simulink model "zadatak3"  (R2017b)
settings: Solver=VariableStepAuto  StartTime=0.0  StopTime=100  FixedStep=0.0001  RelTol=1e-3
settings Model: Creator=Luka  LastModifiedBy=Luka

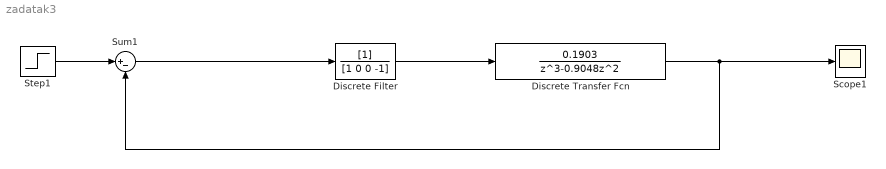
== system zadatak3 ==
  Discrete Transfer Fcn : DiscreteTransferFcn  Numerator=[0.1903]  Denominator=[1 -0.9048 0 0]
  Discrete Filter : DiscreteFilter  Denominator=[1 0 0 -1]
  Scope1 : Scope
  Step1 : Step  Time=0  SampleTime=0
  Sum1 : Sum  Inputs=|+-
  wires:
  Step1/1 -> Sum1/1
  Discrete Transfer Fcn/1 -> Sum1/2, Scope1/1
  Sum1/1 -> Discrete Filter/1
  Discrete Filter/1 -> Discrete Transfer Fcn/1
